simulink model "Modele_Lineaire"  (R2024a)
settings: Solver=VariableStepAuto  StartTime=0.0  StopTime=3  RelTol=1e-3
values from neighbouring files (symbols this model uses):
  den_bille_simu = [7*L_poutre 0]    [Code.m]    (also in Initialisation.m)
  den_mot_simu = [R_m*J_eq  (R_m*B_eq+n_g*n_m*k_m*k_t*K_g.^2)]    [Code.m]    (also in Initialisation.m)
  num_bille_simu = [5*g*r_arm]    [Code.m]    (also in Initialisation.m)
  num_mot_simu = [K_g*n_m*n_g*k_t]    [Code.m]    (also in Initialisation.m)
settings Model: Creator=francoisdesautels  LastModifiedBy=francoisdesautels

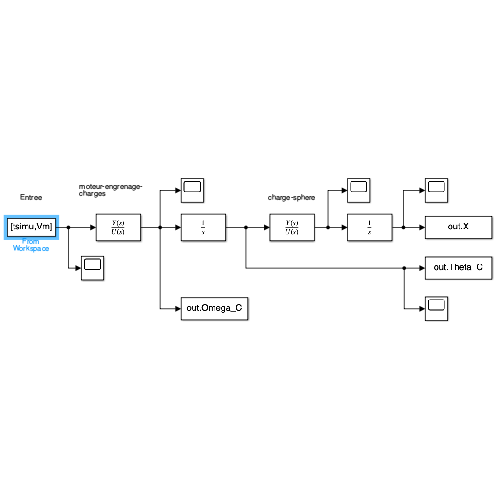
[thumbnail: Simulink's stored preview of the top-level diagram]
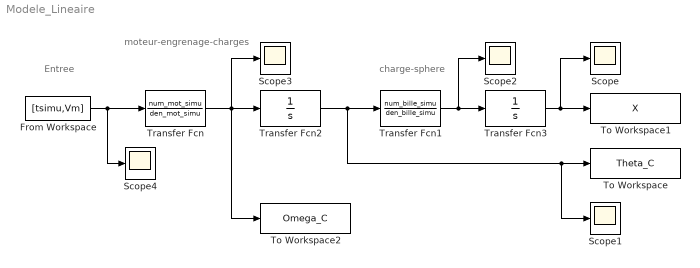
== system Modele_Lineaire ==
  note: charge-sphere
  note: moteur-engrenage-charges
  note: Entree
  From Workspace : FromWorkspace  VariableName=[tsimu,Vm]  SampleTime=-1
  Scope{,1..4} (5 alike) : Scope
  To Workspace : ToWorkspace  VariableName=Theta_C  SaveFormat=Timeseries  SampleTime=-1
      settings: Save2DSignal=2-D array (concatenate along first dimension)
  To Workspace1 : ToWorkspace  VariableName=X  SaveFormat=Timeseries  SampleTime=-1
  To Workspace2 : ToWorkspace  VariableName=Omega_C  SampleTime=-1
  Transfer Fcn : TransferFcn  Numerator=num_mot_simu  Denominator=den_mot_simu
  Transfer Fcn1 : TransferFcn  Numerator=num_bille_simu  Denominator=den_bille_simu
  Transfer Fcn2 : TransferFcn  Denominator=[1 0]
  Transfer Fcn3 : TransferFcn  Denominator=[1 0]
  wires:
  Transfer Fcn/1 -> To Workspace2/1, Scope3/1, Transfer Fcn2/1
  Transfer Fcn1/1 -> Scope2/1, Transfer Fcn3/1
  Transfer Fcn2/1 -> Transfer Fcn1/1, Scope1/1, To Workspace/1
  Transfer Fcn3/1 -> Scope/1, To Workspace1/1
  From Workspace/1 -> Scope4/1, Transfer Fcn/1
